simulink model "IEEE5BusSystemModel_std_UFLS"  (R2019b)
settings: Solver=ode4  StartTime=0.0  StopTime=300  MaxStep=1e-4  RelTol=1e-3
InitFcn:
  | startup_RTS
values from neighbouring files (symbols this model uses):
  C = b/(2*pi*60*Zn)    [startup_RTS.m]
  C0 = C/3    [startup_RTS.m]
  fn = 50    [startup_RTS.m]
  In = Sn/(sqrt(3)*Vn)    [startup_RTS.m]
  L = x*Zn/(2*pi*60)    [startup_RTS.m]
  L0 = 3*L    [startup_RTS.m]
  len = ceil(0.95*300000*T_prop)    [startup_RTS.m]
  PL1 = 300e6    (= 300000000)    [startup_RTS.m]
  PL2 = 300e6    (= 300000000)    [startup_RTS.m]
  PL3 = 300e6    (= 300000000)    [startup_RTS.m]
  QL1 = 30e6    (= 30000000)    [startup_RTS.m]
  QL2 = 30e6    (= 30000000)    [startup_RTS.m]
  QL3 = 30e6    (= 30000000)    [startup_RTS.m]
  R = r*Zn    [startup_RTS.m]
  R0 = 3*R    [startup_RTS.m]
  Sn = 1000e6    (= 1000000000)    [startup_RTS.m]
  t_cont = 100    [startup_RTS.m]
  Vn = 345e3    (= 345000)    [startup_RTS.m]
undefined symbols (not defined in the file or in its folder): D1, Delta
libraries: powerlib x42, powerlib_meascontrol x39, dspswit3 x10, dspstat3 x3, sps_avr x3, spsExcitationSystemModel x3
(part 7 of 7)

== system IEEE5BusSystemModel_std_UFLS/Subsystem5/PMU_e-IpDFT_P-class/Ia_est/Synchrophasor estimation/delta - 2 ==
  X (k max) : Inport
  X (k max + epsilon) : Inport  Port=2
  epsilon : Inport  Port=3
  Abs2 : Abs
  Abs4 : Abs
  Divide : Product  Inputs=*/
  Gain : Gain  Gain=2
  Product : Product  RndMeth=Zero
  Subtract : Sum  Inputs=+-
  Subtract1 : Sum
  delta : Outport  VectorParamsAs1DForOutWhenUnconnected=off
  wires:
  Abs2/1 -> Subtract1/1, Gain/1
  Abs4/1 -> Subtract1/2, Subtract/2
  epsilon/1 -> Product/1
  Product/1 -> delta/1
  Divide/1 -> Product/2
  Subtract1/1 -> Divide/2
  Subtract/1 -> Divide/1
  X (k max + epsilon)/1 -> Abs2/1
  X (k max)/1 -> Abs4/1
  Gain/1 -> Subtract/1

== system IEEE5BusSystemModel_std_UFLS/Subsystem5/PMU_e-IpDFT_P-class/Ia_est/Synchrophasor estimation/epsilon ==
  X (k max -1) : Inport
  X (k max+1) : Inport  Port=2
  Abs1 : Abs
  Abs3 : Abs
  Add5 : Sum  Inputs=+-
  Constant : Constant  SampleTime=Ts_p
  Constant1 : Constant  Value=-1  SampleTime=Ts_p
  Sign : Signum
  Switch : Switch
  Switch1 : Switch  Threshold=1
  X (Kmax + epsilon) : Outport  VectorParamsAs1DForOutWhenUnconnected=off
  epsilon : Outport  Port=2  VectorParamsAs1DForOutWhenUnconnected=off
  wires:
  Constant1/1 -> Switch/3
  Constant/1 -> Switch/1
  Abs1/1 -> Add5/1
  Abs3/1 -> Add5/2
  Sign/1 -> Switch/2
  Add5/1 -> Sign/1
  X (k max -1)/1 -> Abs3/1, Switch1/3
  Switch1/1 -> X (Kmax + epsilon)/1
  Switch/1 -> Switch1/2, epsilon/1
  X (k max+1)/1 -> Abs1/1, Switch1/1

== system IEEE5BusSystemModel_std_UFLS/Subsystem5/PMU_e-IpDFT_P-class/Ia_est/Synchrophasor estimation/spectral leakage compensation ==
  note: xaCORR=2iMAX+dBin
  note: xbCORR=2iMAX+/-1+dBin
  Amplitude : Inport
  delta : Inport  Port=2
  X (k max + epsilon) : Inport  Port=3
  X (k max) : Inport  Port=4
  epsilon : Inport  Port=5
  ph X(k-1) : Inport  Port=6
  Add : Sum
  Add1 : Sum  Inputs=+++
  Complex to Magnitude-Angle1 : ComplexToMagnitudeAngle
  Constant1 : Constant  Value=-1  SampleTime=Ts_p
  Constant3 : Constant  SampleTime=Ts_p
  Constant5 : Constant  Value=pi  SampleTime=Ts_p
  Gain : Gain  Gain=-1
  Gain1 : Gain  Gain=2
  Grandke Magnitude .Correction_A : Subsystem
  Grandke Magnitude .Correction_B : Subsystem
  Magnitude-Angle to Complex : MagnitudeAngleToComplex
  Magnitude-Angle to Complex1 : MagnitudeAngleToComplex
  Subtract1 : Sum  Inputs=+-
  Subtract2 : Sum
  Subtract4 : Sum  Inputs=+-
  Switch1 : Switch  Threshold=1
  Switch3 : Switch  Threshold=1
  Terminator : Terminator
  iMax : Constant  Value=kmax  SampleTime=Inf
  X(k max) : Outport  VectorParamsAs1DForOutWhenUnconnected=off
  X(k max+epsilon) : Outport  Port=2  VectorParamsAs1DForOutWhenUnconnected=off
  wires:
  Gain/1 -> Magnitude-Angle to Complex/2, Magnitude-Angle to Complex1/2
  Add1/1 -> Grandke Magnitude .Correction_B/1(xaCORR)
  Switch3/1 -> Add1/3
  Constant1/1 -> Switch3/3
  Constant3/1 -> Switch3/1
  ph X(k-1)/1 -> Switch1/3
  Complex to Magnitude-Angle1/2 -> Switch1/1
  Gain1/1 -> Add1/2, Add/2
  Grandke Magnitude .Correction_A/1(r CORR) -> Magnitude-Angle to Complex/1
  Add/1 -> Grandke Magnitude .Correction_A/1(xaCORR)
  Grandke Magnitude .Correction_B/1(r CORR) -> Magnitude-Angle to Complex1/1
  Magnitude-Angle to Complex/1 -> Subtract1/2
  Subtract1/1 -> X(k max)/1
  Subtract4/1 -> X(k max+epsilon)/1
  Magnitude-Angle to Complex1/1 -> Subtract4/2
  Amplitude/1 -> Grandke Magnitude .Correction_A/2(Amplitude), Grandke Magnitude .Correction_B/2(Amplitude)
  delta/1 -> Add1/1, Add/1
  X (k max)/1 -> Subtract1/1, Complex to Magnitude-Angle1/1
  epsilon/1 -> Switch3/2, Switch1/2
  Constant5/1 -> Subtract2/2
  Subtract2/1 -> Gain/1
  Switch1/1 -> Subtract2/1
  Complex to Magnitude-Angle1/1 -> Terminator/1
  iMax/1 -> Gain1/1
  X (k max + epsilon)/1 -> Subtract4/1

== system IEEE5BusSystemModel_std_UFLS/Subsystem5/PMU_e-IpDFT_P-class/Ia_est/mSDFT/Kmax ==
  x(n) : Inport
  x(n-M) : Inport  Port=2
  trigger : Inport  Port=3
  2 : Product  RndMeth=Zero
  Conjugate : Math  Operator=conj  SaturateOnIntegerOverflow=on
  Constant : Constant  Value=2/M  SampleTime=Ts_p
  Delay1 : Delay  DelayLength=1  SampleTime=Ts_p
  Delay2 : Delay  DelayLength=1  InitialConditionSource=Input port  ExternalReset=Falling  SampleTime=Ts_p
      settings: InputPortMap=u0,r5,p4
  Product : Product  RndMeth=Zero
  Product1 : Product  RndMeth=Zero
  Product2 : Product  RndMeth=Zero
  Sum : Sum  Inputs=|+-
  Sum1 : Sum  Inputs=|++
  Switch : Switch  Criteria=u2 > Threshold
  imag1 : Constant  Value=Wk(3)  SampleTime=Ts_p
  initialization3 : Constant  Value=1+0*1i  SampleTime=Ts_p
  X(k) : Outport  VectorParamsAs1DForOutWhenUnconnected=off
  wires:
  Switch/1 -> 2/1
  Product2/1 -> Switch/3
  Conjugate/1 -> Product2/2
  Product/1 -> Conjugate/1, Delay2/1
  imag1/1 -> Product/2
  initialization3/1 -> Delay2/3
  Delay2/1 -> Product/1, Product1/2
  trigger/1 -> Switch/2, Delay2/2
  2/1 -> X(k)/1
  Constant/1 -> 2/2
  Sum/1 -> Product1/1
  x(n-M)/1 -> Sum/2
  x(n)/1 -> Sum/1
  Delay1/1 -> Sum1/2
  Sum1/1 -> Product2/1, Switch/1, Delay1/1
  Product1/1 -> Sum1/1

== system IEEE5BusSystemModel_std_UFLS/Subsystem5/PMU_e-IpDFT_P-class/Ia_est/mSDFT/Kmax+1 ==
  x(n) : Inport
  x(n-M) : Inport  Port=2
  trigger : Inport  Port=3
  2 : Product  RndMeth=Zero
  Conjugate : Math  Operator=conj  SaturateOnIntegerOverflow=on
  Constant : Constant  Value=2/M  SampleTime=Ts_p
  Delay1 : Delay  DelayLength=1  SampleTime=Ts_p
  Delay2 : Delay  DelayLength=1  InitialConditionSource=Input port  ExternalReset=Falling  SampleTime=Ts_p
      settings: InputPortMap=u0,r5,p4
  Product : Product  RndMeth=Zero
  Product1 : Product  RndMeth=Zero
  Product2 : Product  RndMeth=Zero
  Sum : Sum  Inputs=|+-
  Sum1 : Sum  Inputs=|++
  Switch : Switch  Criteria=u2 > Threshold
  imag1 : Constant  Value=Wk(4)  SampleTime=Ts_p
  initialization3 : Constant  Value=1+0*1i  SampleTime=Ts_p
  X(k) : Outport  VectorParamsAs1DForOutWhenUnconnected=off
  wires:
  Switch/1 -> 2/1
  Product2/1 -> Switch/3
  Conjugate/1 -> Product2/2
  Product/1 -> Conjugate/1, Delay2/1
  imag1/1 -> Product/2
  initialization3/1 -> Delay2/3
  Delay2/1 -> Product/1, Product1/2
  trigger/1 -> Switch/2, Delay2/2
  2/1 -> X(k)/1
  Constant/1 -> 2/2
  Sum/1 -> Product1/1
  x(n-M)/1 -> Sum/2
  x(n)/1 -> Sum/1
  Delay1/1 -> Sum1/2
  Sum1/1 -> Product2/1, Switch/1, Delay1/1
  Product1/1 -> Sum1/1

== system IEEE5BusSystemModel_std_UFLS/Subsystem5/PMU_e-IpDFT_P-class/Ia_est/mSDFT/Kmax+2 ==
  x(n) : Inport
  x(n-M) : Inport  Port=2
  trigger : Inport  Port=3
  2 : Product  RndMeth=Zero
  Conjugate : Math  Operator=conj  SaturateOnIntegerOverflow=on
  Constant : Constant  Value=2/M  SampleTime=Ts_p
  Delay1 : Delay  DelayLength=1  SampleTime=Ts_p
  Delay2 : Delay  DelayLength=1  InitialConditionSource=Input port  ExternalReset=Falling  SampleTime=Ts_p
      settings: InputPortMap=u0,r5,p4
  Product : Product  RndMeth=Zero
  Product1 : Product  RndMeth=Zero
  Product2 : Product  RndMeth=Zero
  Sum : Sum  Inputs=|+-
  Sum1 : Sum  Inputs=|++
  Switch : Switch  Criteria=u2 > Threshold
  imag1 : Constant  Value=Wk(5)  SampleTime=Ts_p
  initialization3 : Constant  Value=1+0*1i  SampleTime=Ts_p
  X(k) : Outport  VectorParamsAs1DForOutWhenUnconnected=off
  wires:
  Switch/1 -> 2/1
  Product2/1 -> Switch/3
  Conjugate/1 -> Product2/2
  Product/1 -> Conjugate/1, Delay2/1
  imag1/1 -> Product/2
  initialization3/1 -> Delay2/3
  Delay2/1 -> Product/1, Product1/2
  trigger/1 -> Switch/2, Delay2/2
  2/1 -> X(k)/1
  Constant/1 -> 2/2
  Sum/1 -> Product1/1
  x(n-M)/1 -> Sum/2
  x(n)/1 -> Sum/1
  Delay1/1 -> Sum1/2
  Sum1/1 -> Product2/1, Switch/1, Delay1/1
  Product1/1 -> Sum1/1

== system IEEE5BusSystemModel_std_UFLS/Subsystem5/PMU_e-IpDFT_P-class/Ia_est/mSDFT/Kmax-1 ==
  x(n) : Inport
  x(n-M) : Inport  Port=2
  trigger : Inport  Port=3
  2 : Product  RndMeth=Zero
  Conjugate : Math  Operator=conj  SaturateOnIntegerOverflow=on
  Constant : Constant  Value=2/M  SampleTime=Ts_p
  Delay1 : Delay  DelayLength=1  SampleTime=Ts_p
  Delay2 : Delay  DelayLength=1  InitialConditionSource=Input port  ExternalReset=Falling  SampleTime=Ts_p
      settings: InputPortMap=u0,r5,p4
  Product : Product  RndMeth=Zero
  Product1 : Product  RndMeth=Zero
  Product2 : Product  RndMeth=Zero
  Sum : Sum  Inputs=|+-
  Sum1 : Sum  Inputs=|++
  Switch : Switch  Criteria=u2 > Threshold
  imag1 : Constant  Value=Wk(2)  SampleTime=Ts_p
  initialization3 : Constant  Value=1+0*1i  SampleTime=Ts_p
  X(k) : Outport  VectorParamsAs1DForOutWhenUnconnected=off
  wires:
  Switch/1 -> 2/1
  Product2/1 -> Switch/3
  Conjugate/1 -> Product2/2
  Product/1 -> Conjugate/1, Delay2/1
  imag1/1 -> Product/2
  initialization3/1 -> Delay2/3
  Delay2/1 -> Product/1, Product1/2
  trigger/1 -> Switch/2, Delay2/2
  2/1 -> X(k)/1
  Constant/1 -> 2/2
  Sum/1 -> Product1/1
  x(n-M)/1 -> Sum/2
  x(n)/1 -> Sum/1
  Delay1/1 -> Sum1/2
  Sum1/1 -> Product2/1, Switch/1, Delay1/1
  Product1/1 -> Sum1/1

== system IEEE5BusSystemModel_std_UFLS/Subsystem5/PMU_e-IpDFT_P-class/Ia_est/mSDFT/Kmax-2 ==
  x(n) : Inport
  x(n-M) : Inport  Port=2
  trigger : Inport  Port=3
  2 : Product  RndMeth=Zero
  Conjugate : Math  Operator=conj  SaturateOnIntegerOverflow=on
  Constant : Constant  Value=2/M  SampleTime=Ts_p
  Delay1 : Delay  DelayLength=1  SampleTime=Ts_p
  Delay2 : Delay  DelayLength=1  InitialConditionSource=Input port  ExternalReset=Falling  SampleTime=Ts_p
      settings: InputPortMap=u0,r5,p4
  Product : Product  RndMeth=Zero
  Product1 : Product  RndMeth=Zero
  Product2 : Product  RndMeth=Zero
  Sum : Sum  Inputs=|+-
  Sum1 : Sum  Inputs=|++
  Switch : Switch  Criteria=u2 > Threshold
  imag1 : Constant  Value=Wk(1)  SampleTime=Ts_p
  initialization3 : Constant  Value=1+0*1i  SampleTime=Ts_p
  X(k) : Outport  VectorParamsAs1DForOutWhenUnconnected=off
  wires:
  Switch/1 -> 2/1
  Product2/1 -> Switch/3
  Conjugate/1 -> Product2/2
  Product/1 -> Conjugate/1, Delay2/1
  imag1/1 -> Product/2
  initialization3/1 -> Delay2/3
  Delay2/1 -> Product/1, Product1/2
  trigger/1 -> Switch/2, Delay2/2
  2/1 -> X(k)/1
  Constant/1 -> 2/2
  Sum/1 -> Product1/1
  x(n-M)/1 -> Sum/2
  x(n)/1 -> Sum/1
  Delay1/1 -> Sum1/2
  Sum1/1 -> Product2/1, Switch/1, Delay1/1
  Product1/1 -> Sum1/1

== system IEEE5BusSystemModel_std_UFLS/Subsystem5/PMU_e-IpDFT_P-class1/Ia_est/Synchrophasor estimation/Amplitude - 1 ==
  delta : Inport
  (X k_max) : Inport  Port=2
  Abs1 : Abs
  Abs2 : Abs
  Abs3 : Abs
  Constant : Constant  SampleTime=Ts_p
  Constant2 : Constant  SampleTime=Ts_p
  Fcn1 : Fcn  Expr=(pi*u)/sin(pi*u)
  Gain : Gain  Gain=-1
  Product : Product  RndMeth=Zero
  Product2 : Product  Inputs=3  RndMeth=Zero
  Sum : Sum  Inputs=|++
  Switch1 : Switch  Criteria=u2 ~= 0
  amplitude : Outport  VectorParamsAs1DForOutWhenUnconnected=off
  wires:
  Abs2/1 -> Product2/1
  Product/1 -> Gain/1
  Sum/1 -> Product2/3
  Constant/1 -> Sum/2
  Abs1/1 -> Product2/2
  Switch1/1 -> Abs2/1
  Constant2/1 -> Switch1/3
  Abs3/1 -> Switch1/2
  Fcn1/1 -> Switch1/1
  (X k_max)/1 -> Abs1/1
  Product2/1 -> amplitude/1
  delta/1 -> Product/1, Product/2, Abs3/1, Fcn1/1
  Gain/1 -> Sum/1

== system IEEE5BusSystemModel_std_UFLS/Subsystem5/PMU_e-IpDFT_P-class1/Ia_est/Synchrophasor estimation/Amplitude - 2 ==
  delta : Inport
  (X k_max) : Inport  Port=2
  Abs1 : Abs
  Abs2 : Abs
  Abs3 : Abs
  Constant : Constant  SampleTime=Inf
  Constant2 : Constant  SampleTime=Ts_p
  Fcn1 : Fcn  Expr=(pi*u)/sin(pi*u)
  Gain : Gain  Gain=-1
  Gain1 : Gain  Gain=sqrt(2)
  Product : Product  RndMeth=Zero
  Product2 : Product  Inputs=3  RndMeth=Zero
  Sum : Sum  Inputs=|++
  Switch1 : Switch  Criteria=u2 ~= 0
  amplitude : Outport  VectorParamsAs1DForOutWhenUnconnected=off
  wires:
  Abs2/1 -> Product2/1
  Product/1 -> Gain/1
  Sum/1 -> Product2/3
  Constant/1 -> Sum/2
  Abs1/1 -> Product2/2
  Switch1/1 -> Abs2/1
  Constant2/1 -> Switch1/3
  Abs3/1 -> Switch1/2
  Fcn1/1 -> Switch1/1
  (X k_max)/1 -> Abs1/1
  Product2/1 -> Gain1/1
  delta/1 -> Product/1, Product/2, Abs3/1, Fcn1/1
  Gain/1 -> Sum/1
  Gain1/1 -> amplitude/1

== system IEEE5BusSystemModel_std_UFLS/Subsystem5/PMU_e-IpDFT_P-class1/Ia_est/Synchrophasor estimation/Frequency - 2 ==
  delta : Inport
  dF [Hz] : Inport  Port=2
  Add : Sum
  Constant1 : Constant  Value=kmax  SampleTime=Ts_p
  Product : Product  RndMeth=Zero
  frequency : Outport  VectorParamsAs1DForOutWhenUnconnected=off
  wires:
  Add/1 -> Product/2
  Constant1/1 -> Add/1
  delta/1 -> Add/2
  Product/1 -> frequency/1
  dF [Hz]/1 -> Product/1

== system IEEE5BusSystemModel_std_UFLS/Subsystem5/PMU_e-IpDFT_P-class1/Ia_est/Synchrophasor estimation/Hanning(Kmax) ==
  Kmax-1 : Inport
  Kmax : Inport  Port=2
  Kmax+1 : Inport  Port=3
  Add1 : Sum  Inputs=+++
  Constant3 : Constant  Value=-0.25  SampleTime=Ts_p
  Constant4 : Constant  Value=0.5  SampleTime=Ts_p
  Constant5 : Constant  Value=-0.25  SampleTime=Ts_p
  Product3 : Product  RndMeth=Zero
  Product4 : Product  RndMeth=Zero
  Product5 : Product  RndMeth=Zero
  Hanning out : Outport  VectorParamsAs1DForOutWhenUnconnected=off
  wires:
  Add1/1 -> Hanning out/1
  Kmax+1/1 -> Product5/1
  Kmax/1 -> Product4/1
  Kmax-1/1 -> Product3/1
  Product5/1 -> Add1/3
  Product4/1 -> Add1/2
  Product3/1 -> Add1/1
  Constant4/1 -> Product4/2
  Constant5/1 -> Product5/2
  Constant3/1 -> Product3/2

== system IEEE5BusSystemModel_std_UFLS/Subsystem5/PMU_e-IpDFT_P-class1/Ia_est/Synchrophasor estimation/Hanning(Kmax+1) ==
  Kmax : Inport
  Kmax+1 : Inport  Port=2
  Kmax+2 : Inport  Port=3
  Add2 : Sum  Inputs=+++
  Constant6 : Constant  Value=-0.25  SampleTime=Ts_p
  Constant7 : Constant  Value=0.5  SampleTime=Ts_p
  Constant8 : Constant  Value=-0.25  SampleTime=Ts_p
  Product6 : Product  RndMeth=Zero
  Product7 : Product  RndMeth=Zero
  Product8 : Product  RndMeth=Zero
  Hanning out : Outport  VectorParamsAs1DForOutWhenUnconnected=off
  wires:
  Kmax+2/1 -> Product8/1
  Add2/1 -> Hanning out/1
  Kmax+1/1 -> Product7/1
  Kmax/1 -> Product6/1
  Product8/1 -> Add2/3
  Product7/1 -> Add2/2
  Product6/1 -> Add2/1
  Constant7/1 -> Product7/2
  Constant8/1 -> Product8/2
  Constant6/1 -> Product6/2

== system IEEE5BusSystemModel_std_UFLS/Subsystem5/PMU_e-IpDFT_P-class1/Ia_est/Synchrophasor estimation/Hanning(Kmax-1) ==
  Kmax-2 : Inport
  Kmax-1 : Inport  Port=2
  Kmax : Inport  Port=3
  Add : Sum  Inputs=+++
  Constant : Constant  Value=-0.25  SampleTime=Ts_p
  Constant1 : Constant  Value=0.5  SampleTime=Ts_p
  Constant2 : Constant  Value=-0.25  SampleTime=Ts_p
  Product : Product  RndMeth=Zero
  Product1 : Product  RndMeth=Zero
  Product2 : Product  RndMeth=Zero
  Hanning out : Outport  VectorParamsAs1DForOutWhenUnconnected=off
  wires:
  Add/1 -> Hanning out/1
  Kmax-2/1 -> Product/1
  Kmax/1 -> Product2/1
  Kmax-1/1 -> Product1/1
  Product2/1 -> Add/3
  Product1/1 -> Add/2
  Product/1 -> Add/1
  Constant1/1 -> Product1/2
  Constant2/1 -> Product2/2
  Constant/1 -> Product/2

== system IEEE5BusSystemModel_std_UFLS/Subsystem5/PMU_e-IpDFT_P-class1/Ia_est/Synchrophasor estimation/Phase - 2 ==
  X k_max phase : Inport
  delta : Inport  Port=2
  freq : Inport  Port=3
  dT [s] : Inport  Port=4
  Add1 : Sum  Inputs=+-
  Add3 : Sum  Inputs=+++
  Constant3 : Constant  Value=pi  SampleTime=Ts_p
  Constant5 : Constant  Value=2*pi  SampleTime=Ts_p
  Gain : Gain  Gain=2*pi*T/2
  Product : Product  RndMeth=Zero
  Product1 : Product  Inputs=3  RndMeth=Zero
  WrapToPi : Subsystem
  phase : Outport  VectorParamsAs1DForOutWhenUnconnected=off
  wires:
  Product1/1 -> Add3/3
  Gain/1 -> Add3/2
  Add3/1 -> WrapToPi/1(angle in)
  Add1/1 -> Add3/1
  WrapToPi/1(angle out) -> phase/1
  freq/1 -> Gain/1, Product1/1
  dT [s]/1 -> Product1/3
  Constant5/1 -> Product1/2
  Product/1 -> Add1/2
  delta/1 -> Product/1
  X k_max phase/1 -> Add1/1
  Constant3/1 -> Product/2

== system IEEE5BusSystemModel_std_UFLS/Subsystem5/PMU_e-IpDFT_P-class1/Ia_est/Synchrophasor estimation/delta - 1  ==
  X (k max) : Inport
  X (k max + epsilon) : Inport  Port=2
  epsilon : Inport  Port=3
  Abs2 : Abs
  Abs4 : Abs
  Divide : Product  Inputs=*/
  Gain : Gain  Gain=2
  Product : Product  RndMeth=Zero
  Subtract : Sum  Inputs=+-
  Subtract1 : Sum
  delta : Outport  VectorParamsAs1DForOutWhenUnconnected=off
  wires:
  epsilon/1 -> Product/1
  Product/1 -> delta/1
  Divide/1 -> Product/2
  Subtract1/1 -> Divide/2
  Subtract/1 -> Divide/1
  X (k max + epsilon)/1 -> Abs2/1
  X (k max)/1 -> Abs4/1
  Gain/1 -> Subtract/1
  Abs4/1 -> Subtract1/2, Subtract/2
  Abs2/1 -> Subtract1/1, Gain/1

== system IEEE5BusSystemModel_std_UFLS/Subsystem5/PMU_e-IpDFT_P-class1/Ia_est/Synchrophasor estimation/delta - 2 ==
  X (k max) : Inport
  X (k max + epsilon) : Inport  Port=2
  epsilon : Inport  Port=3
  Abs2 : Abs
  Abs4 : Abs
  Divide : Product  Inputs=*/
  Gain : Gain  Gain=2
  Product : Product  RndMeth=Zero
  Subtract : Sum  Inputs=+-
  Subtract1 : Sum
  delta : Outport  VectorParamsAs1DForOutWhenUnconnected=off
  wires:
  Gain/1 -> Subtract/1
  X (k max)/1 -> Abs4/1
  X (k max + epsilon)/1 -> Abs2/1
  Subtract/1 -> Divide/1
  Subtract1/1 -> Divide/2
  Divide/1 -> Product/2
  Product/1 -> delta/1
  epsilon/1 -> Product/1
  Abs4/1 -> Subtract/2, Subtract1/2
  Abs2/1 -> Gain/1, Subtract1/1

== system IEEE5BusSystemModel_std_UFLS/Subsystem5/PMU_e-IpDFT_P-class1/Ia_est/Synchrophasor estimation/epsilon ==
  X (k max -1) : Inport
  X (k max+1) : Inport  Port=2
  Abs1 : Abs
  Abs3 : Abs
  Add5 : Sum  Inputs=+-
  Constant : Constant  SampleTime=Ts_p
  Constant1 : Constant  Value=-1  SampleTime=Ts_p
  Sign : Signum
  Switch : Switch
  Switch1 : Switch  Threshold=1
  X (Kmax + epsilon) : Outport  VectorParamsAs1DForOutWhenUnconnected=off
  epsilon : Outport  Port=2  VectorParamsAs1DForOutWhenUnconnected=off
  wires:
  X (k max+1)/1 -> Switch1/1, Abs1/1
  Switch/1 -> epsilon/1, Switch1/2
  Switch1/1 -> X (Kmax + epsilon)/1
  X (k max -1)/1 -> Switch1/3, Abs3/1
  Add5/1 -> Sign/1
  Sign/1 -> Switch/2
  Abs3/1 -> Add5/2
  Abs1/1 -> Add5/1
  Constant/1 -> Switch/1
  Constant1/1 -> Switch/3

== system IEEE5BusSystemModel_std_UFLS/Subsystem5/PMU_e-IpDFT_P-class1/Ia_est/Synchrophasor estimation/spectral leakage compensation ==
  note: xbCORR=2iMAX+/-1+dBin
  note: xaCORR=2iMAX+dBin
  Amplitude : Inport
  delta : Inport  Port=2
  X (k max + epsilon) : Inport  Port=3
  X (k max) : Inport  Port=4
  epsilon : Inport  Port=5
  ph X(k-1) : Inport  Port=6
  Add : Sum
  Add1 : Sum  Inputs=+++
  Complex to Magnitude-Angle1 : ComplexToMagnitudeAngle
  Constant1 : Constant  Value=-1  SampleTime=Ts_p
  Constant3 : Constant  SampleTime=Ts_p
  Constant5 : Constant  Value=pi  SampleTime=Ts_p
  Gain : Gain  Gain=-1
  Gain1 : Gain  Gain=2
  Grandke Magnitude .Correction_A : Subsystem
  Grandke Magnitude .Correction_B : Subsystem
  Magnitude-Angle to Complex : MagnitudeAngleToComplex
  Magnitude-Angle to Complex1 : MagnitudeAngleToComplex
  Subtract1 : Sum  Inputs=+-
  Subtract2 : Sum
  Subtract4 : Sum  Inputs=+-
  Switch1 : Switch  Threshold=1
  Switch3 : Switch  Threshold=1
  Terminator : Terminator
  iMax : Constant  Value=kmax  SampleTime=Inf
  X(k max) : Outport  VectorParamsAs1DForOutWhenUnconnected=off
  X(k max+epsilon) : Outport  Port=2  VectorParamsAs1DForOutWhenUnconnected=off
  wires:
  X (k max + epsilon)/1 -> Subtract4/1
  iMax/1 -> Gain1/1
  Complex to Magnitude-Angle1/1 -> Terminator/1
  Switch1/1 -> Subtract2/1
  Subtract2/1 -> Gain/1
  Constant5/1 -> Subtract2/2
  epsilon/1 -> Switch1/2, Switch3/2
  X (k max)/1 -> Complex to Magnitude-Angle1/1, Subtract1/1
  delta/1 -> Add/1, Add1/1
  Amplitude/1 -> Grandke Magnitude .Correction_B/2(Amplitude), Grandke Magnitude .Correction_A/2(Amplitude)
  Magnitude-Angle to Complex1/1 -> Subtract4/2
  Subtract4/1 -> X(k max+epsilon)/1
  Subtract1/1 -> X(k max)/1
  Magnitude-Angle to Complex/1 -> Subtract1/2
  Grandke Magnitude .Correction_B/1(r CORR) -> Magnitude-Angle to Complex1/1
  Add/1 -> Grandke Magnitude .Correction_A/1(xaCORR)
  Grandke Magnitude .Correction_A/1(r CORR) -> Magnitude-Angle to Complex/1
  Gain1/1 -> Add/2, Add1/2
  Complex to Magnitude-Angle1/2 -> Switch1/1
  ph X(k-1)/1 -> Switch1/3
  Constant3/1 -> Switch3/1
  Constant1/1 -> Switch3/3
  Switch3/1 -> Add1/3
  Add1/1 -> Grandke Magnitude .Correction_B/1(xaCORR)
  Gain/1 -> Magnitude-Angle to Complex1/2, Magnitude-Angle to Complex/2

== system IEEE5BusSystemModel_std_UFLS/Subsystem5/PMU_e-IpDFT_P-class1/Ia_est/mSDFT/Kmax ==
  x(n) : Inport
  x(n-M) : Inport  Port=2
  trigger : Inport  Port=3
  2 : Product  RndMeth=Zero
  Conjugate : Math  Operator=conj  SaturateOnIntegerOverflow=on
  Constant : Constant  Value=2/M  SampleTime=Ts_p
  Delay1 : Delay  DelayLength=1  SampleTime=Ts_p
  Delay2 : Delay  DelayLength=1  InitialConditionSource=Input port  ExternalReset=Falling  SampleTime=Ts_p
      settings: InputPortMap=u0,r5,p4
  Product : Product  RndMeth=Zero
  Product1 : Product  RndMeth=Zero
  Product2 : Product  RndMeth=Zero
  Sum : Sum  Inputs=|+-
  Sum1 : Sum  Inputs=|++
  Switch : Switch  Criteria=u2 > Threshold
  imag1 : Constant  Value=Wk(3)  SampleTime=Ts_p
  initialization3 : Constant  Value=1+0*1i  SampleTime=Ts_p
  X(k) : Outport  VectorParamsAs1DForOutWhenUnconnected=off
  wires:
  Product1/1 -> Sum1/1
  Sum1/1 -> Delay1/1, Switch/1, Product2/1
  Delay1/1 -> Sum1/2
  x(n)/1 -> Sum/1
  x(n-M)/1 -> Sum/2
  Sum/1 -> Product1/1
  Constant/1 -> 2/2
  2/1 -> X(k)/1
  trigger/1 -> Delay2/2, Switch/2
  Delay2/1 -> Product1/2, Product/1
  initialization3/1 -> Delay2/3
  imag1/1 -> Product/2
  Product/1 -> Delay2/1, Conjugate/1
  Conjugate/1 -> Product2/2
  Product2/1 -> Switch/3
  Switch/1 -> 2/1

== system IEEE5BusSystemModel_std_UFLS/Subsystem5/PMU_e-IpDFT_P-class1/Ia_est/mSDFT/Kmax+1 ==
  x(n) : Inport
  x(n-M) : Inport  Port=2
  trigger : Inport  Port=3
  2 : Product  RndMeth=Zero
  Conjugate : Math  Operator=conj  SaturateOnIntegerOverflow=on
  Constant : Constant  Value=2/M  SampleTime=Ts_p
  Delay1 : Delay  DelayLength=1  SampleTime=Ts_p
  Delay2 : Delay  DelayLength=1  InitialConditionSource=Input port  ExternalReset=Falling  SampleTime=Ts_p
      settings: InputPortMap=u0,r5,p4
  Product : Product  RndMeth=Zero
  Product1 : Product  RndMeth=Zero
  Product2 : Product  RndMeth=Zero
  Sum : Sum  Inputs=|+-
  Sum1 : Sum  Inputs=|++
  Switch : Switch  Criteria=u2 > Threshold
  imag1 : Constant  Value=Wk(4)  SampleTime=Ts_p
  initialization3 : Constant  Value=1+0*1i  SampleTime=Ts_p
  X(k) : Outport  VectorParamsAs1DForOutWhenUnconnected=off
  wires:
  Product1/1 -> Sum1/1
  Sum1/1 -> Delay1/1, Switch/1, Product2/1
  Delay1/1 -> Sum1/2
  x(n)/1 -> Sum/1
  x(n-M)/1 -> Sum/2
  Sum/1 -> Product1/1
  Constant/1 -> 2/2
  2/1 -> X(k)/1
  trigger/1 -> Delay2/2, Switch/2
  Delay2/1 -> Product1/2, Product/1
  initialization3/1 -> Delay2/3
  imag1/1 -> Product/2
  Product/1 -> Delay2/1, Conjugate/1
  Conjugate/1 -> Product2/2
  Product2/1 -> Switch/3
  Switch/1 -> 2/1

== system IEEE5BusSystemModel_std_UFLS/Subsystem5/PMU_e-IpDFT_P-class1/Ia_est/mSDFT/Kmax+2 ==
  x(n) : Inport
  x(n-M) : Inport  Port=2
  trigger : Inport  Port=3
  2 : Product  RndMeth=Zero
  Conjugate : Math  Operator=conj  SaturateOnIntegerOverflow=on
  Constant : Constant  Value=2/M  SampleTime=Ts_p
  Delay1 : Delay  DelayLength=1  SampleTime=Ts_p
  Delay2 : Delay  DelayLength=1  InitialConditionSource=Input port  ExternalReset=Falling  SampleTime=Ts_p
      settings: InputPortMap=u0,r5,p4
  Product : Product  RndMeth=Zero
  Product1 : Product  RndMeth=Zero
  Product2 : Product  RndMeth=Zero
  Sum : Sum  Inputs=|+-
  Sum1 : Sum  Inputs=|++
  Switch : Switch  Criteria=u2 > Threshold
  imag1 : Constant  Value=Wk(5)  SampleTime=Ts_p
  initialization3 : Constant  Value=1+0*1i  SampleTime=Ts_p
  X(k) : Outport  VectorParamsAs1DForOutWhenUnconnected=off
  wires:
  Product1/1 -> Sum1/1
  Sum1/1 -> Delay1/1, Switch/1, Product2/1
  Delay1/1 -> Sum1/2
  x(n)/1 -> Sum/1
  x(n-M)/1 -> Sum/2
  Sum/1 -> Product1/1
  Constant/1 -> 2/2
  2/1 -> X(k)/1
  trigger/1 -> Delay2/2, Switch/2
  Delay2/1 -> Product1/2, Product/1
  initialization3/1 -> Delay2/3
  imag1/1 -> Product/2
  Product/1 -> Delay2/1, Conjugate/1
  Conjugate/1 -> Product2/2
  Product2/1 -> Switch/3
  Switch/1 -> 2/1

== system IEEE5BusSystemModel_std_UFLS/Subsystem5/PMU_e-IpDFT_P-class1/Ia_est/mSDFT/Kmax-1 ==
  x(n) : Inport
  x(n-M) : Inport  Port=2
  trigger : Inport  Port=3
  2 : Product  RndMeth=Zero
  Conjugate : Math  Operator=conj  SaturateOnIntegerOverflow=on
  Constant : Constant  Value=2/M  SampleTime=Ts_p
  Delay1 : Delay  DelayLength=1  SampleTime=Ts_p
  Delay2 : Delay  DelayLength=1  InitialConditionSource=Input port  ExternalReset=Falling  SampleTime=Ts_p
      settings: InputPortMap=u0,r5,p4
  Product : Product  RndMeth=Zero
  Product1 : Product  RndMeth=Zero
  Product2 : Product  RndMeth=Zero
  Sum : Sum  Inputs=|+-
  Sum1 : Sum  Inputs=|++
  Switch : Switch  Criteria=u2 > Threshold
  imag1 : Constant  Value=Wk(2)  SampleTime=Ts_p
  initialization3 : Constant  Value=1+0*1i  SampleTime=Ts_p
  X(k) : Outport  VectorParamsAs1DForOutWhenUnconnected=off
  wires:
  Product1/1 -> Sum1/1
  Sum1/1 -> Delay1/1, Switch/1, Product2/1
  Delay1/1 -> Sum1/2
  x(n)/1 -> Sum/1
  x(n-M)/1 -> Sum/2
  Sum/1 -> Product1/1
  Constant/1 -> 2/2
  2/1 -> X(k)/1
  trigger/1 -> Delay2/2, Switch/2
  Delay2/1 -> Product1/2, Product/1
  initialization3/1 -> Delay2/3
  imag1/1 -> Product/2
  Product/1 -> Delay2/1, Conjugate/1
  Conjugate/1 -> Product2/2
  Product2/1 -> Switch/3
  Switch/1 -> 2/1

== system IEEE5BusSystemModel_std_UFLS/Subsystem5/PMU_e-IpDFT_P-class1/Ia_est/mSDFT/Kmax-2 ==
  x(n) : Inport
  x(n-M) : Inport  Port=2
  trigger : Inport  Port=3
  2 : Product  RndMeth=Zero
  Conjugate : Math  Operator=conj  SaturateOnIntegerOverflow=on
  Constant : Constant  Value=2/M  SampleTime=Ts_p
  Delay1 : Delay  DelayLength=1  SampleTime=Ts_p
  Delay2 : Delay  DelayLength=1  InitialConditionSource=Input port  ExternalReset=Falling  SampleTime=Ts_p
      settings: InputPortMap=u0,r5,p4
  Product : Product  RndMeth=Zero
  Product1 : Product  RndMeth=Zero
  Product2 : Product  RndMeth=Zero
  Sum : Sum  Inputs=|+-
  Sum1 : Sum  Inputs=|++
  Switch : Switch  Criteria=u2 > Threshold
  imag1 : Constant  Value=Wk(1)  SampleTime=Ts_p
  initialization3 : Constant  Value=1+0*1i  SampleTime=Ts_p
  X(k) : Outport  VectorParamsAs1DForOutWhenUnconnected=off
  wires:
  Product1/1 -> Sum1/1
  Sum1/1 -> Delay1/1, Switch/1, Product2/1
  Delay1/1 -> Sum1/2
  x(n)/1 -> Sum/1
  x(n-M)/1 -> Sum/2
  Sum/1 -> Product1/1
  Constant/1 -> 2/2
  2/1 -> X(k)/1
  trigger/1 -> Delay2/2, Switch/2
  Delay2/1 -> Product1/2, Product/1
  initialization3/1 -> Delay2/3
  imag1/1 -> Product/2
  Product/1 -> Delay2/1, Conjugate/1
  Conjugate/1 -> Product2/2
  Product2/1 -> Switch/3
  Switch/1 -> 2/1

== system IEEE5BusSystemModel_std_UFLS/Subsystem1/PMU_e-IpDFT_P-class/Ia_est/Synchrophasor estimation/Phase - 2/WrapToPi ==
  angle in : Inport
  Constant12 : Constant  Value=2*pi  SampleTime=Inf
  Constant13 : Constant  Value=pi  SampleTime=Inf
  Constant14 : Constant  Value=pi  SampleTime=Inf
  Math Function5 : Math  Operator=mod  SaturateOnIntegerOverflow=on
  Sum1 : Sum  Inputs=|++
  Sum2 : Sum  Inputs=|+-
  angle out : Outport  VectorParamsAs1DForOutWhenUnconnected=off
  wires:
  Sum2/1 -> angle out/1
  angle in/1 -> Sum1/1
  Constant14/1 -> Sum2/2
  Math Function5/1 -> Sum2/1
  Constant13/1 -> Sum1/2
  Sum1/1 -> Math Function5/1
  Constant12/1 -> Math Function5/2

== system IEEE5BusSystemModel_std_UFLS/Subsystem1/PMU_e-IpDFT_P-class/Ia_est/Synchrophasor estimation/spectral leakage compensation/Grandke Magnitude .Correction_A ==
  xaCORR : Inport
  Amplitude : Inport  Port=2
  Abs1 : Abs
  Constant1 : Constant  SampleTime=Ts_p
  Divide : Product  Inputs=*/
  Fcn1 : Fcn  Expr=sin(pi*u)/(pi*u)
  Math Function : Math  Operator=square  SaturateOnIntegerOverflow=on
  Product6 : Product  RndMeth=Zero
  Sum : Sum  Inputs=|+-
  r CORR : Outport  VectorParamsAs1DForOutWhenUnconnected=off
  wires:
  Divide/1 -> Abs1/1
  Sum/1 -> Divide/2
  Math Function/1 -> Sum/1
  xaCORR/1 -> Math Function/1, Fcn1/1
  Amplitude/1 -> Product6/1
  Product6/1 -> r CORR/1
  Fcn1/1 -> Divide/1
  Constant1/1 -> Sum/2
  Abs1/1 -> Product6/2

== system IEEE5BusSystemModel_std_UFLS/Subsystem1/PMU_e-IpDFT_P-class/Ia_est/Synchrophasor estimation/spectral leakage compensation/Grandke Magnitude .Correction_B ==
  xaCORR : Inport
  Amplitude : Inport  Port=2
  Abs1 : Abs
  Constant1 : Constant  SampleTime=Ts_p
  Divide : Product  Inputs=*/
  Fcn1 : Fcn  Expr=sin(pi*u)/(pi*u)
  Math Function : Math  Operator=square  SaturateOnIntegerOverflow=on
  Product6 : Product  RndMeth=Zero
  Sum : Sum  Inputs=|+-
  r CORR : Outport  VectorParamsAs1DForOutWhenUnconnected=off
  wires:
  Divide/1 -> Abs1/1
  Sum/1 -> Divide/2
  Math Function/1 -> Sum/1
  xaCORR/1 -> Math Function/1, Fcn1/1
  Amplitude/1 -> Product6/1
  Product6/1 -> r CORR/1
  Fcn1/1 -> Divide/1
  Constant1/1 -> Sum/2
  Abs1/1 -> Product6/2

== system IEEE5BusSystemModel_std_UFLS/Subsystem1/PMU_e-IpDFT_P-class1/Ia_est/Synchrophasor estimation/Phase - 2/WrapToPi ==
  angle in : Inport
  Constant12 : Constant  Value=2*pi  SampleTime=Inf
  Constant13 : Constant  Value=pi  SampleTime=Inf
  Constant14 : Constant  Value=pi  SampleTime=Inf
  Math Function5 : Math  Operator=mod  SaturateOnIntegerOverflow=on
  Sum1 : Sum  Inputs=|++
  Sum2 : Sum  Inputs=|+-
  angle out : Outport  VectorParamsAs1DForOutWhenUnconnected=off
  wires:
  Constant12/1 -> Math Function5/2
  Sum1/1 -> Math Function5/1
  Constant13/1 -> Sum1/2
  Math Function5/1 -> Sum2/1
  Constant14/1 -> Sum2/2
  angle in/1 -> Sum1/1
  Sum2/1 -> angle out/1

== system IEEE5BusSystemModel_std_UFLS/Subsystem1/PMU_e-IpDFT_P-class1/Ia_est/Synchrophasor estimation/spectral leakage compensation/Grandke Magnitude .Correction_A ==
  xaCORR : Inport
  Amplitude : Inport  Port=2
  Abs1 : Abs
  Constant1 : Constant  SampleTime=Ts_p
  Divide : Product  Inputs=*/
  Fcn1 : Fcn  Expr=sin(pi*u)/(pi*u)
  Math Function : Math  Operator=square  SaturateOnIntegerOverflow=on
  Product6 : Product  RndMeth=Zero
  Sum : Sum  Inputs=|+-
  r CORR : Outport  VectorParamsAs1DForOutWhenUnconnected=off
  wires:
  Abs1/1 -> Product6/2
  Constant1/1 -> Sum/2
  Fcn1/1 -> Divide/1
  Product6/1 -> r CORR/1
  Amplitude/1 -> Product6/1
  xaCORR/1 -> Fcn1/1, Math Function/1
  Math Function/1 -> Sum/1
  Sum/1 -> Divide/2
  Divide/1 -> Abs1/1

== system IEEE5BusSystemModel_std_UFLS/Subsystem1/PMU_e-IpDFT_P-class1/Ia_est/Synchrophasor estimation/spectral leakage compensation/Grandke Magnitude .Correction_B ==
  xaCORR : Inport
  Amplitude : Inport  Port=2
  Abs1 : Abs
  Constant1 : Constant  SampleTime=Ts_p
  Divide : Product  Inputs=*/
  Fcn1 : Fcn  Expr=sin(pi*u)/(pi*u)
  Math Function : Math  Operator=square  SaturateOnIntegerOverflow=on
  Product6 : Product  RndMeth=Zero
  Sum : Sum  Inputs=|+-
  r CORR : Outport  VectorParamsAs1DForOutWhenUnconnected=off
  wires:
  Abs1/1 -> Product6/2
  Constant1/1 -> Sum/2
  Fcn1/1 -> Divide/1
  Product6/1 -> r CORR/1
  Amplitude/1 -> Product6/1
  xaCORR/1 -> Fcn1/1, Math Function/1
  Math Function/1 -> Sum/1
  Sum/1 -> Divide/2
  Divide/1 -> Abs1/1

== system IEEE5BusSystemModel_std_UFLS/Subsystem2/PMU_e-IpDFT_P-class/Ia_est/Synchrophasor estimation/Phase - 2/WrapToPi ==
  angle in : Inport
  Constant12 : Constant  Value=2*pi  SampleTime=Inf
  Constant13 : Constant  Value=pi  SampleTime=Inf
  Constant14 : Constant  Value=pi  SampleTime=Inf
  Math Function5 : Math  Operator=mod  SaturateOnIntegerOverflow=on
  Sum1 : Sum  Inputs=|++
  Sum2 : Sum  Inputs=|+-
  angle out : Outport  VectorParamsAs1DForOutWhenUnconnected=off
  wires:
  Constant12/1 -> Math Function5/2
  Sum1/1 -> Math Function5/1
  Constant13/1 -> Sum1/2
  Math Function5/1 -> Sum2/1
  Constant14/1 -> Sum2/2
  angle in/1 -> Sum1/1
  Sum2/1 -> angle out/1

== system IEEE5BusSystemModel_std_UFLS/Subsystem2/PMU_e-IpDFT_P-class/Ia_est/Synchrophasor estimation/spectral leakage compensation/Grandke Magnitude .Correction_A ==
  xaCORR : Inport
  Amplitude : Inport  Port=2
  Abs1 : Abs
  Constant1 : Constant  SampleTime=Ts_p
  Divide : Product  Inputs=*/
  Fcn1 : Fcn  Expr=sin(pi*u)/(pi*u)
  Math Function : Math  Operator=square  SaturateOnIntegerOverflow=on
  Product6 : Product  RndMeth=Zero
  Sum : Sum  Inputs=|+-
  r CORR : Outport  VectorParamsAs1DForOutWhenUnconnected=off
  wires:
  Abs1/1 -> Product6/2
  Constant1/1 -> Sum/2
  Fcn1/1 -> Divide/1
  Product6/1 -> r CORR/1
  Amplitude/1 -> Product6/1
  xaCORR/1 -> Fcn1/1, Math Function/1
  Math Function/1 -> Sum/1
  Sum/1 -> Divide/2
  Divide/1 -> Abs1/1

== system IEEE5BusSystemModel_std_UFLS/Subsystem2/PMU_e-IpDFT_P-class/Ia_est/Synchrophasor estimation/spectral leakage compensation/Grandke Magnitude .Correction_B ==
  xaCORR : Inport
  Amplitude : Inport  Port=2
  Abs1 : Abs
  Constant1 : Constant  SampleTime=Ts_p
  Divide : Product  Inputs=*/
  Fcn1 : Fcn  Expr=sin(pi*u)/(pi*u)
  Math Function : Math  Operator=square  SaturateOnIntegerOverflow=on
  Product6 : Product  RndMeth=Zero
  Sum : Sum  Inputs=|+-
  r CORR : Outport  VectorParamsAs1DForOutWhenUnconnected=off
  wires:
  Abs1/1 -> Product6/2
  Constant1/1 -> Sum/2
  Fcn1/1 -> Divide/1
  Product6/1 -> r CORR/1
  Amplitude/1 -> Product6/1
  xaCORR/1 -> Fcn1/1, Math Function/1
  Math Function/1 -> Sum/1
  Sum/1 -> Divide/2
  Divide/1 -> Abs1/1

== system IEEE5BusSystemModel_std_UFLS/Subsystem2/PMU_e-IpDFT_P-class1/Ia_est/Synchrophasor estimation/Phase - 2/WrapToPi ==
  angle in : Inport
  Constant12 : Constant  Value=2*pi  SampleTime=Inf
  Constant13 : Constant  Value=pi  SampleTime=Inf
  Constant14 : Constant  Value=pi  SampleTime=Inf
  Math Function5 : Math  Operator=mod  SaturateOnIntegerOverflow=on
  Sum1 : Sum  Inputs=|++
  Sum2 : Sum  Inputs=|+-
  angle out : Outport  VectorParamsAs1DForOutWhenUnconnected=off
  wires:
  Sum2/1 -> angle out/1
  angle in/1 -> Sum1/1
  Constant14/1 -> Sum2/2
  Math Function5/1 -> Sum2/1
  Constant13/1 -> Sum1/2
  Sum1/1 -> Math Function5/1
  Constant12/1 -> Math Function5/2

== system IEEE5BusSystemModel_std_UFLS/Subsystem2/PMU_e-IpDFT_P-class1/Ia_est/Synchrophasor estimation/spectral leakage compensation/Grandke Magnitude .Correction_A ==
  xaCORR : Inport
  Amplitude : Inport  Port=2
  Abs1 : Abs
  Constant1 : Constant  SampleTime=Ts_p
  Divide : Product  Inputs=*/
  Fcn1 : Fcn  Expr=sin(pi*u)/(pi*u)
  Math Function : Math  Operator=square  SaturateOnIntegerOverflow=on
  Product6 : Product  RndMeth=Zero
  Sum : Sum  Inputs=|+-
  r CORR : Outport  VectorParamsAs1DForOutWhenUnconnected=off
  wires:
  Divide/1 -> Abs1/1
  Sum/1 -> Divide/2
  Math Function/1 -> Sum/1
  xaCORR/1 -> Math Function/1, Fcn1/1
  Amplitude/1 -> Product6/1
  Product6/1 -> r CORR/1
  Fcn1/1 -> Divide/1
  Constant1/1 -> Sum/2
  Abs1/1 -> Product6/2

== system IEEE5BusSystemModel_std_UFLS/Subsystem2/PMU_e-IpDFT_P-class1/Ia_est/Synchrophasor estimation/spectral leakage compensation/Grandke Magnitude .Correction_B ==
  xaCORR : Inport
  Amplitude : Inport  Port=2
  Abs1 : Abs
  Constant1 : Constant  SampleTime=Ts_p
  Divide : Product  Inputs=*/
  Fcn1 : Fcn  Expr=sin(pi*u)/(pi*u)
  Math Function : Math  Operator=square  SaturateOnIntegerOverflow=on
  Product6 : Product  RndMeth=Zero
  Sum : Sum  Inputs=|+-
  r CORR : Outport  VectorParamsAs1DForOutWhenUnconnected=off
  wires:
  Divide/1 -> Abs1/1
  Sum/1 -> Divide/2
  Math Function/1 -> Sum/1
  xaCORR/1 -> Math Function/1, Fcn1/1
  Amplitude/1 -> Product6/1
  Product6/1 -> r CORR/1
  Fcn1/1 -> Divide/1
  Constant1/1 -> Sum/2
  Abs1/1 -> Product6/2

== system IEEE5BusSystemModel_std_UFLS/Subsystem3/PMU_e-IpDFT_P-class/Ia_est/Synchrophasor estimation/Phase - 2/WrapToPi ==
  angle in : Inport
  Constant12 : Constant  Value=2*pi  SampleTime=Inf
  Constant13 : Constant  Value=pi  SampleTime=Inf
  Constant14 : Constant  Value=pi  SampleTime=Inf
  Math Function5 : Math  Operator=mod  SaturateOnIntegerOverflow=on
  Sum1 : Sum  Inputs=|++
  Sum2 : Sum  Inputs=|+-
  angle out : Outport  VectorParamsAs1DForOutWhenUnconnected=off
  wires:
  Sum2/1 -> angle out/1
  angle in/1 -> Sum1/1
  Constant14/1 -> Sum2/2
  Math Function5/1 -> Sum2/1
  Constant13/1 -> Sum1/2
  Sum1/1 -> Math Function5/1
  Constant12/1 -> Math Function5/2

== system IEEE5BusSystemModel_std_UFLS/Subsystem3/PMU_e-IpDFT_P-class/Ia_est/Synchrophasor estimation/spectral leakage compensation/Grandke Magnitude .Correction_A ==
  xaCORR : Inport
  Amplitude : Inport  Port=2
  Abs1 : Abs
  Constant1 : Constant  SampleTime=Ts_p
  Divide : Product  Inputs=*/
  Fcn1 : Fcn  Expr=sin(pi*u)/(pi*u)
  Math Function : Math  Operator=square  SaturateOnIntegerOverflow=on
  Product6 : Product  RndMeth=Zero
  Sum : Sum  Inputs=|+-
  r CORR : Outport  VectorParamsAs1DForOutWhenUnconnected=off
  wires:
  Divide/1 -> Abs1/1
  Sum/1 -> Divide/2
  Math Function/1 -> Sum/1
  xaCORR/1 -> Math Function/1, Fcn1/1
  Amplitude/1 -> Product6/1
  Product6/1 -> r CORR/1
  Fcn1/1 -> Divide/1
  Constant1/1 -> Sum/2
  Abs1/1 -> Product6/2

== system IEEE5BusSystemModel_std_UFLS/Subsystem3/PMU_e-IpDFT_P-class/Ia_est/Synchrophasor estimation/spectral leakage compensation/Grandke Magnitude .Correction_B ==
  xaCORR : Inport
  Amplitude : Inport  Port=2
  Abs1 : Abs
  Constant1 : Constant  SampleTime=Ts_p
  Divide : Product  Inputs=*/
  Fcn1 : Fcn  Expr=sin(pi*u)/(pi*u)
  Math Function : Math  Operator=square  SaturateOnIntegerOverflow=on
  Product6 : Product  RndMeth=Zero
  Sum : Sum  Inputs=|+-
  r CORR : Outport  VectorParamsAs1DForOutWhenUnconnected=off
  wires:
  Divide/1 -> Abs1/1
  Sum/1 -> Divide/2
  Math Function/1 -> Sum/1
  xaCORR/1 -> Math Function/1, Fcn1/1
  Amplitude/1 -> Product6/1
  Product6/1 -> r CORR/1
  Fcn1/1 -> Divide/1
  Constant1/1 -> Sum/2
  Abs1/1 -> Product6/2

== system IEEE5BusSystemModel_std_UFLS/Subsystem3/PMU_e-IpDFT_P-class1/Ia_est/Synchrophasor estimation/Phase - 2/WrapToPi ==
  angle in : Inport
  Constant12 : Constant  Value=2*pi  SampleTime=Inf
  Constant13 : Constant  Value=pi  SampleTime=Inf
  Constant14 : Constant  Value=pi  SampleTime=Inf
  Math Function5 : Math  Operator=mod  SaturateOnIntegerOverflow=on
  Sum1 : Sum  Inputs=|++
  Sum2 : Sum  Inputs=|+-
  angle out : Outport  VectorParamsAs1DForOutWhenUnconnected=off
  wires:
  Constant12/1 -> Math Function5/2
  Sum1/1 -> Math Function5/1
  Constant13/1 -> Sum1/2
  Math Function5/1 -> Sum2/1
  Constant14/1 -> Sum2/2
  angle in/1 -> Sum1/1
  Sum2/1 -> angle out/1

== system IEEE5BusSystemModel_std_UFLS/Subsystem3/PMU_e-IpDFT_P-class1/Ia_est/Synchrophasor estimation/spectral leakage compensation/Grandke Magnitude .Correction_A ==
  xaCORR : Inport
  Amplitude : Inport  Port=2
  Abs1 : Abs
  Constant1 : Constant  SampleTime=Ts_p
  Divide : Product  Inputs=*/
  Fcn1 : Fcn  Expr=sin(pi*u)/(pi*u)
  Math Function : Math  Operator=square  SaturateOnIntegerOverflow=on
  Product6 : Product  RndMeth=Zero
  Sum : Sum  Inputs=|+-
  r CORR : Outport  VectorParamsAs1DForOutWhenUnconnected=off
  wires:
  Abs1/1 -> Product6/2
  Constant1/1 -> Sum/2
  Fcn1/1 -> Divide/1
  Product6/1 -> r CORR/1
  Amplitude/1 -> Product6/1
  xaCORR/1 -> Fcn1/1, Math Function/1
  Math Function/1 -> Sum/1
  Sum/1 -> Divide/2
  Divide/1 -> Abs1/1

== system IEEE5BusSystemModel_std_UFLS/Subsystem3/PMU_e-IpDFT_P-class1/Ia_est/Synchrophasor estimation/spectral leakage compensation/Grandke Magnitude .Correction_B ==
  xaCORR : Inport
  Amplitude : Inport  Port=2
  Abs1 : Abs
  Constant1 : Constant  SampleTime=Ts_p
  Divide : Product  Inputs=*/
  Fcn1 : Fcn  Expr=sin(pi*u)/(pi*u)
  Math Function : Math  Operator=square  SaturateOnIntegerOverflow=on
  Product6 : Product  RndMeth=Zero
  Sum : Sum  Inputs=|+-
  r CORR : Outport  VectorParamsAs1DForOutWhenUnconnected=off
  wires:
  Abs1/1 -> Product6/2
  Constant1/1 -> Sum/2
  Fcn1/1 -> Divide/1
  Product6/1 -> r CORR/1
  Amplitude/1 -> Product6/1
  xaCORR/1 -> Fcn1/1, Math Function/1
  Math Function/1 -> Sum/1
  Sum/1 -> Divide/2
  Divide/1 -> Abs1/1

== system IEEE5BusSystemModel_std_UFLS/Subsystem4/PMU_e-IpDFT_P-class/Ia_est/Synchrophasor estimation/Phase - 2/WrapToPi ==
  angle in : Inport
  Constant12 : Constant  Value=2*pi  SampleTime=Inf
  Constant13 : Constant  Value=pi  SampleTime=Inf
  Constant14 : Constant  Value=pi  SampleTime=Inf
  Math Function5 : Math  Operator=mod  SaturateOnIntegerOverflow=on
  Sum1 : Sum  Inputs=|++
  Sum2 : Sum  Inputs=|+-
  angle out : Outport  VectorParamsAs1DForOutWhenUnconnected=off
  wires:
  Constant12/1 -> Math Function5/2
  Sum1/1 -> Math Function5/1
  Constant13/1 -> Sum1/2
  Math Function5/1 -> Sum2/1
  Constant14/1 -> Sum2/2
  angle in/1 -> Sum1/1
  Sum2/1 -> angle out/1

== system IEEE5BusSystemModel_std_UFLS/Subsystem4/PMU_e-IpDFT_P-class/Ia_est/Synchrophasor estimation/spectral leakage compensation/Grandke Magnitude .Correction_A ==
  xaCORR : Inport
  Amplitude : Inport  Port=2
  Abs1 : Abs
  Constant1 : Constant  SampleTime=Ts_p
  Divide : Product  Inputs=*/
  Fcn1 : Fcn  Expr=sin(pi*u)/(pi*u)
  Math Function : Math  Operator=square  SaturateOnIntegerOverflow=on
  Product6 : Product  RndMeth=Zero
  Sum : Sum  Inputs=|+-
  r CORR : Outport  VectorParamsAs1DForOutWhenUnconnected=off
  wires:
  Abs1/1 -> Product6/2
  Constant1/1 -> Sum/2
  Fcn1/1 -> Divide/1
  Product6/1 -> r CORR/1
  Amplitude/1 -> Product6/1
  xaCORR/1 -> Fcn1/1, Math Function/1
  Math Function/1 -> Sum/1
  Sum/1 -> Divide/2
  Divide/1 -> Abs1/1

== system IEEE5BusSystemModel_std_UFLS/Subsystem4/PMU_e-IpDFT_P-class/Ia_est/Synchrophasor estimation/spectral leakage compensation/Grandke Magnitude .Correction_B ==
  xaCORR : Inport
  Amplitude : Inport  Port=2
  Abs1 : Abs
  Constant1 : Constant  SampleTime=Ts_p
  Divide : Product  Inputs=*/
  Fcn1 : Fcn  Expr=sin(pi*u)/(pi*u)
  Math Function : Math  Operator=square  SaturateOnIntegerOverflow=on
  Product6 : Product  RndMeth=Zero
  Sum : Sum  Inputs=|+-
  r CORR : Outport  VectorParamsAs1DForOutWhenUnconnected=off
  wires:
  Abs1/1 -> Product6/2
  Constant1/1 -> Sum/2
  Fcn1/1 -> Divide/1
  Product6/1 -> r CORR/1
  Amplitude/1 -> Product6/1
  xaCORR/1 -> Fcn1/1, Math Function/1
  Math Function/1 -> Sum/1
  Sum/1 -> Divide/2
  Divide/1 -> Abs1/1

== system IEEE5BusSystemModel_std_UFLS/Subsystem4/PMU_e-IpDFT_P-class1/Ia_est/Synchrophasor estimation/Phase - 2/WrapToPi ==
  angle in : Inport
  Constant12 : Constant  Value=2*pi  SampleTime=Inf
  Constant13 : Constant  Value=pi  SampleTime=Inf
  Constant14 : Constant  Value=pi  SampleTime=Inf
  Math Function5 : Math  Operator=mod  SaturateOnIntegerOverflow=on
  Sum1 : Sum  Inputs=|++
  Sum2 : Sum  Inputs=|+-
  angle out : Outport  VectorParamsAs1DForOutWhenUnconnected=off
  wires:
  Sum2/1 -> angle out/1
  angle in/1 -> Sum1/1
  Constant14/1 -> Sum2/2
  Math Function5/1 -> Sum2/1
  Constant13/1 -> Sum1/2
  Sum1/1 -> Math Function5/1
  Constant12/1 -> Math Function5/2

== system IEEE5BusSystemModel_std_UFLS/Subsystem4/PMU_e-IpDFT_P-class1/Ia_est/Synchrophasor estimation/spectral leakage compensation/Grandke Magnitude .Correction_A ==
  xaCORR : Inport
  Amplitude : Inport  Port=2
  Abs1 : Abs
  Constant1 : Constant  SampleTime=Ts_p
  Divide : Product  Inputs=*/
  Fcn1 : Fcn  Expr=sin(pi*u)/(pi*u)
  Math Function : Math  Operator=square  SaturateOnIntegerOverflow=on
  Product6 : Product  RndMeth=Zero
  Sum : Sum  Inputs=|+-
  r CORR : Outport  VectorParamsAs1DForOutWhenUnconnected=off
  wires:
  Divide/1 -> Abs1/1
  Sum/1 -> Divide/2
  Math Function/1 -> Sum/1
  xaCORR/1 -> Math Function/1, Fcn1/1
  Amplitude/1 -> Product6/1
  Product6/1 -> r CORR/1
  Fcn1/1 -> Divide/1
  Constant1/1 -> Sum/2
  Abs1/1 -> Product6/2

== system IEEE5BusSystemModel_std_UFLS/Subsystem4/PMU_e-IpDFT_P-class1/Ia_est/Synchrophasor estimation/spectral leakage compensation/Grandke Magnitude .Correction_B ==
  xaCORR : Inport
  Amplitude : Inport  Port=2
  Abs1 : Abs
  Constant1 : Constant  SampleTime=Ts_p
  Divide : Product  Inputs=*/
  Fcn1 : Fcn  Expr=sin(pi*u)/(pi*u)
  Math Function : Math  Operator=square  SaturateOnIntegerOverflow=on
  Product6 : Product  RndMeth=Zero
  Sum : Sum  Inputs=|+-
  r CORR : Outport  VectorParamsAs1DForOutWhenUnconnected=off
  wires:
  Divide/1 -> Abs1/1
  Sum/1 -> Divide/2
  Math Function/1 -> Sum/1
  xaCORR/1 -> Math Function/1, Fcn1/1
  Amplitude/1 -> Product6/1
  Product6/1 -> r CORR/1
  Fcn1/1 -> Divide/1
  Constant1/1 -> Sum/2
  Abs1/1 -> Product6/2

== system IEEE5BusSystemModel_std_UFLS/Subsystem5/PMU_e-IpDFT_P-class/Ia_est/Synchrophasor estimation/Phase - 2/WrapToPi ==
  angle in : Inport
  Constant12 : Constant  Value=2*pi  SampleTime=Inf
  Constant13 : Constant  Value=pi  SampleTime=Inf
  Constant14 : Constant  Value=pi  SampleTime=Inf
  Math Function5 : Math  Operator=mod  SaturateOnIntegerOverflow=on
  Sum1 : Sum  Inputs=|++
  Sum2 : Sum  Inputs=|+-
  angle out : Outport  VectorParamsAs1DForOutWhenUnconnected=off
  wires:
  Constant12/1 -> Math Function5/2
  Sum1/1 -> Math Function5/1
  Constant13/1 -> Sum1/2
  Math Function5/1 -> Sum2/1
  Constant14/1 -> Sum2/2
  angle in/1 -> Sum1/1
  Sum2/1 -> angle out/1

== system IEEE5BusSystemModel_std_UFLS/Subsystem5/PMU_e-IpDFT_P-class/Ia_est/Synchrophasor estimation/spectral leakage compensation/Grandke Magnitude .Correction_A ==
  xaCORR : Inport
  Amplitude : Inport  Port=2
  Abs1 : Abs
  Constant1 : Constant  SampleTime=Ts_p
  Divide : Product  Inputs=*/
  Fcn1 : Fcn  Expr=sin(pi*u)/(pi*u)
  Math Function : Math  Operator=square  SaturateOnIntegerOverflow=on
  Product6 : Product  RndMeth=Zero
  Sum : Sum  Inputs=|+-
  r CORR : Outport  VectorParamsAs1DForOutWhenUnconnected=off
  wires:
  Abs1/1 -> Product6/2
  Constant1/1 -> Sum/2
  Fcn1/1 -> Divide/1
  Product6/1 -> r CORR/1
  Amplitude/1 -> Product6/1
  xaCORR/1 -> Fcn1/1, Math Function/1
  Math Function/1 -> Sum/1
  Sum/1 -> Divide/2
  Divide/1 -> Abs1/1

== system IEEE5BusSystemModel_std_UFLS/Subsystem5/PMU_e-IpDFT_P-class/Ia_est/Synchrophasor estimation/spectral leakage compensation/Grandke Magnitude .Correction_B ==
  xaCORR : Inport
  Amplitude : Inport  Port=2
  Abs1 : Abs
  Constant1 : Constant  SampleTime=Ts_p
  Divide : Product  Inputs=*/
  Fcn1 : Fcn  Expr=sin(pi*u)/(pi*u)
  Math Function : Math  Operator=square  SaturateOnIntegerOverflow=on
  Product6 : Product  RndMeth=Zero
  Sum : Sum  Inputs=|+-
  r CORR : Outport  VectorParamsAs1DForOutWhenUnconnected=off
  wires:
  Abs1/1 -> Product6/2
  Constant1/1 -> Sum/2
  Fcn1/1 -> Divide/1
  Product6/1 -> r CORR/1
  Amplitude/1 -> Product6/1
  xaCORR/1 -> Fcn1/1, Math Function/1
  Math Function/1 -> Sum/1
  Sum/1 -> Divide/2
  Divide/1 -> Abs1/1

== system IEEE5BusSystemModel_std_UFLS/Subsystem5/PMU_e-IpDFT_P-class1/Ia_est/Synchrophasor estimation/Phase - 2/WrapToPi ==
  angle in : Inport
  Constant12 : Constant  Value=2*pi  SampleTime=Inf
  Constant13 : Constant  Value=pi  SampleTime=Inf
  Constant14 : Constant  Value=pi  SampleTime=Inf
  Math Function5 : Math  Operator=mod  SaturateOnIntegerOverflow=on
  Sum1 : Sum  Inputs=|++
  Sum2 : Sum  Inputs=|+-
  angle out : Outport  VectorParamsAs1DForOutWhenUnconnected=off
  wires:
  Sum2/1 -> angle out/1
  angle in/1 -> Sum1/1
  Constant14/1 -> Sum2/2
  Math Function5/1 -> Sum2/1
  Constant13/1 -> Sum1/2
  Sum1/1 -> Math Function5/1
  Constant12/1 -> Math Function5/2

== system IEEE5BusSystemModel_std_UFLS/Subsystem5/PMU_e-IpDFT_P-class1/Ia_est/Synchrophasor estimation/spectral leakage compensation/Grandke Magnitude .Correction_A ==
  xaCORR : Inport
  Amplitude : Inport  Port=2
  Abs1 : Abs
  Constant1 : Constant  SampleTime=Ts_p
  Divide : Product  Inputs=*/
  Fcn1 : Fcn  Expr=sin(pi*u)/(pi*u)
  Math Function : Math  Operator=square  SaturateOnIntegerOverflow=on
  Product6 : Product  RndMeth=Zero
  Sum : Sum  Inputs=|+-
  r CORR : Outport  VectorParamsAs1DForOutWhenUnconnected=off
  wires:
  Divide/1 -> Abs1/1
  Sum/1 -> Divide/2
  Math Function/1 -> Sum/1
  xaCORR/1 -> Math Function/1, Fcn1/1
  Amplitude/1 -> Product6/1
  Product6/1 -> r CORR/1
  Fcn1/1 -> Divide/1
  Constant1/1 -> Sum/2
  Abs1/1 -> Product6/2

== system IEEE5BusSystemModel_std_UFLS/Subsystem5/PMU_e-IpDFT_P-class1/Ia_est/Synchrophasor estimation/spectral leakage compensation/Grandke Magnitude .Correction_B ==
  xaCORR : Inport
  Amplitude : Inport  Port=2
  Abs1 : Abs
  Constant1 : Constant  SampleTime=Ts_p
  Divide : Product  Inputs=*/
  Fcn1 : Fcn  Expr=sin(pi*u)/(pi*u)
  Math Function : Math  Operator=square  SaturateOnIntegerOverflow=on
  Product6 : Product  RndMeth=Zero
  Sum : Sum  Inputs=|+-
  r CORR : Outport  VectorParamsAs1DForOutWhenUnconnected=off
  wires:
  Divide/1 -> Abs1/1
  Sum/1 -> Divide/2
  Math Function/1 -> Sum/1
  xaCORR/1 -> Math Function/1, Fcn1/1
  Amplitude/1 -> Product6/1
  Product6/1 -> r CORR/1
  Fcn1/1 -> Divide/1
  Constant1/1 -> Sum/2
  Abs1/1 -> Product6/2
